simulink model "current_controller"  (R2015a)
settings: Solver=ode45  StartTime=0.0  StopTime=10.0  RelTol=1e-3
values from neighbouring files (symbols this model uses):
  Em = 115*sqrt(2)    [current_controller_param.m]
  Idref = 3    [current_controller_param.m]
  Iqref = 0    [current_controller_param.m]
  Kii = alphaI*R_hat    (= 628.318530718)    [VOC_param_paper.m]    (also in controller_parameters.m; current_controller_param.m = 1260)
  Kpi = alphaI*L_hat    (= 37.6991118431)    [VOC_param_paper.m]    (also in controller_parameters.m; current_controller_param.m = 62.8)
  L = 8e-3    (= 0.008)    [VOC_param.m]    (also in VOC_param_paper.m = 0.003; controller_parameters.m = 0.003; current_controller_param.m = 0.005; power_control_param.m)
  R = 0.1    [VOC_param.m]    (also in VOC_param_paper.m = 0.05; controller_parameters.m = 0.05; current_controller_param.m; power_control_param.m)
  w = 2*pi*f    (= 314.159265359)    [VOC_param.m]    (also in controller_parameters.m; current_controller_param.m; power_control_param.m)
libraries: powerlib_meascontrol x2, simulink x2
settings Model: Creator=rblan  LastModifiedBy=rblan

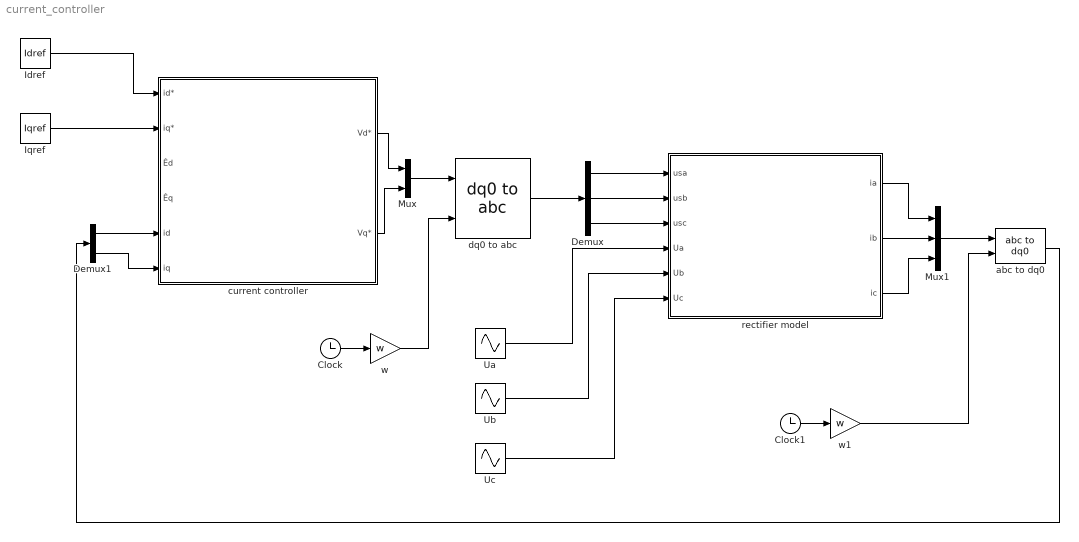
== system current_controller ==
  Clock : Clock
  Clock1 : Clock
  Demux : Demux  Outputs=3
  Demux1 : Demux  Outputs=2
  Idref : Constant  Value=Idref
  Iqref : Constant  Value=Iqref
  Mux : Mux  Inputs=2
  Mux1 : Mux  Inputs=3
  Ua : Sin  Amplitude=Em  Frequency=w  SampleTime=0
  Ub : Sin  Amplitude=Em  Frequency=w  Phase=-2*pi*3  SampleTime=0
  Uc : Sin  Amplitude=Em  Frequency=w  Phase=-4*pi/3  SampleTime=0
  abc to dq0 : powerlib_meascontrol/Transformations/abc to dq0  Alignment=90 degrees behind phase A axis
  "current controller " : Subsystem
  dq0 to abc : powerlib_meascontrol/Transformations/dq0 to abc  Alignment=90 degrees behind phase A axis
  rectifier model : Subsystem
  w : Gain  Gain=w
  w1 : Gain  Gain=w
  wires:
  "current controller "/1(Vd*) -> Mux/1
  "current controller "/2(Vq*) -> Mux/2
  Mux/1 -> dq0 to abc/1
  dq0 to abc/1 -> Demux/1
  Demux/1 -> rectifier model/1(usa)
  Demux/2 -> rectifier model/2(usb)
  Demux/3 -> rectifier model/3(usc)
  rectifier model/1(ia) -> Mux1/1
  rectifier model/2(ib) -> Mux1/2
  rectifier model/3(ic) -> Mux1/3
  Mux1/1 -> abc to dq0/1
  Demux1/2 -> "current controller "/6(iq)
  Demux1/1 -> "current controller "/5(id)
  abc to dq0/1 -> Demux1/1
  Ua/1 -> rectifier model/4(Ua)
  Ub/1 -> rectifier model/5(Ub)
  Uc/1 -> rectifier model/6(Uc)
  Idref/1 -> "current controller "/1(id*)
  Iqref/1 -> "current controller "/2(iq*)
  Clock/1 -> w/1
  w/1 -> dq0 to abc/2
  Clock1/1 -> w1/1
  w1/1 -> abc to dq0/2

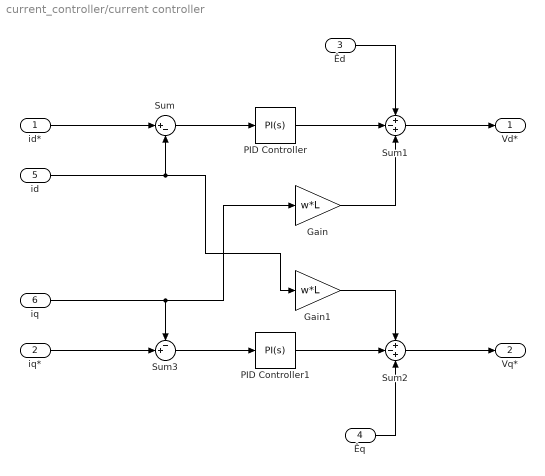
== system current_controller/current controller  ==
  id* : Inport
  iq* : Inport  Port=2
  Êd : Inport  Port=3
  Êq : Inport  Port=4
  id : Inport  Port=5
  iq : Inport  Port=6
  Gain : Gain  Gain=w*L
  Gain1 : Gain  Gain=w*L
  PID Controller : simulink/Continuous/PID Controller  Controller=PI  TimeDomain=Continuous-time  SampleTime=-1  IntegratorMethod=Forward Euler  FilterMethod=Forward Euler  Form=Parallel  UseFilter=on  ControllerParametersSource=internal  P=Kpi  I=Kii  D=0  N=100  InitialConditionSource=internal  InitialConditionForIntegrator=0  InitialConditionForFilter=0  ExternalReset=none  LimitOutput=off  UpperSaturationLimit=inf  LowerSaturationLimit=-inf  LinearizeAsGain=on  AntiWindupMode=none  Kb=1  TrackingMode=off  Kt=1  PParamMin=[]  PParamMax=[]  IParamMin=[]  IParamMax=[]  DParamMin=[]  DParamMax=[]  NParamMin=[]  NParamMax=[]  KbParamMin=[]  KbParamMax=[]  KtParamMin=[]  KtParamMax=[]  POutMin=[]  POutMax=[]  IOutMin=[]  IOutMax=[]  DOutMin=[]  DOutMax=[]  NOutMin=[]  NOutMax=[]  KbOutMin=[]  KbOutMax=[]  KtOutMin=[]  KtOutMax=[]  IntegratorOutMin=[]  IntegratorOutMax=[]  FilterOutMin=[]  FilterOutMax=[]  SumOutMin=[]  SumOutMax=[]  SumI1OutMin=[]  SumI1OutMax=[]  SumI2OutMin=[]  SumI2OutMax=[]  SumI3OutMin=[]  SumI3OutMax=[]  SumDOutMin=[]  SumDOutMax=[]  SaturationOutMin=[]  SaturationOutMax=[]  IntegratorContinuousStateAttributes=''  IntegratorStateMustResolveToSignalObject=off  IntegratorRTWStateStorageClass=Auto  FilterContinuousStateAttributes=''  FilterStateMustResolveToSignalObject=off  FilterRTWStateStorageClass=Auto  DifferentiatorICPrevScaledInput=0  DifferentiatorOutMin=[]  DifferentiatorOutMax=[]
  PID Controller1 : simulink/Continuous/PID Controller  Controller=PI  TimeDomain=Continuous-time  SampleTime=-1  IntegratorMethod=Forward Euler  FilterMethod=Forward Euler  Form=Parallel  UseFilter=on  ControllerParametersSource=internal  P=Kpi  I=Kii  D=0  N=100  InitialConditionSource=internal  InitialConditionForIntegrator=0  InitialConditionForFilter=0  ExternalReset=none  LimitOutput=off  UpperSaturationLimit=inf  LowerSaturationLimit=-inf  LinearizeAsGain=on  AntiWindupMode=none  Kb=1  TrackingMode=off  Kt=1  PParamMin=[]  PParamMax=[]  IParamMin=[]  IParamMax=[]  DParamMin=[]  DParamMax=[]  NParamMin=[]  NParamMax=[]  KbParamMin=[]  KbParamMax=[]  KtParamMin=[]  KtParamMax=[]  POutMin=[]  POutMax=[]  IOutMin=[]  IOutMax=[]  DOutMin=[]  DOutMax=[]  NOutMin=[]  NOutMax=[]  KbOutMin=[]  KbOutMax=[]  KtOutMin=[]  KtOutMax=[]  IntegratorOutMin=[]  IntegratorOutMax=[]  FilterOutMin=[]  FilterOutMax=[]  SumOutMin=[]  SumOutMax=[]  SumI1OutMin=[]  SumI1OutMax=[]  SumI2OutMin=[]  SumI2OutMax=[]  SumI3OutMin=[]  SumI3OutMax=[]  SumDOutMin=[]  SumDOutMax=[]  SaturationOutMin=[]  SaturationOutMax=[]  IntegratorContinuousStateAttributes=''  IntegratorStateMustResolveToSignalObject=off  IntegratorRTWStateStorageClass=Auto  FilterContinuousStateAttributes=''  FilterStateMustResolveToSignalObject=off  FilterRTWStateStorageClass=Auto  DifferentiatorICPrevScaledInput=0  DifferentiatorOutMin=[]  DifferentiatorOutMax=[]
  Sum : Sum  Inputs=|+-
  Sum1 : Sum  Inputs=+-+
  Sum2 : Sum  Inputs=+-+
  Sum3 : Sum  Inputs=-+|
  Vd* : Outport
  Vq* : Outport  Port=2
  wires:
  id*/1 -> Sum/1
  Sum/1 -> PID Controller/1
  PID Controller/1 -> Sum1/2
  Êd/1 -> Sum1/1
  Sum1/1 -> Vd*/1
  PID Controller1/1 -> Sum2/2
  Sum2/1 -> Vq*/1
  Êq/1 -> Sum2/3
  Sum3/1 -> PID Controller1/1
  iq*/1 -> Sum3/2
  id/1 -> Sum/2, Gain1/1
  iq/1 -> Gain/1, Sum3/1
  Gain/1 -> Sum1/3
  Gain1/1 -> Sum2/1

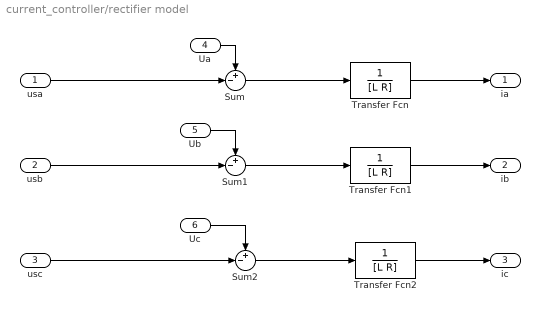
== system current_controller/rectifier model ==
  usa : Inport
  usb : Inport  Port=2
  usc : Inport  Port=3
  Ua : Inport  Port=4
  Ub : Inport  Port=5
  Uc : Inport  Port=6
  Sum : Sum  Inputs=+-|
  Sum1 : Sum  Inputs=+-|
  Sum2 : Sum  Inputs=+-|
  Transfer Fcn : TransferFcn  Denominator=[L R]
  Transfer Fcn1 : TransferFcn  Denominator=[L R]
  Transfer Fcn2 : TransferFcn  Denominator=[L R]
  ia : Outport
  ib : Outport  Port=2
  ic : Outport  Port=3
  wires:
  usa/1 -> Sum/2
  usc/1 -> Sum2/2
  Ua/1 -> Sum/1
  usb/1 -> Sum1/2
  Ub/1 -> Sum1/1
  Uc/1 -> Sum2/1
  Sum/1 -> Transfer Fcn/1
  Sum2/1 -> Transfer Fcn2/1
  Transfer Fcn/1 -> ia/1
  Transfer Fcn1/1 -> ib/1
  Sum1/1 -> Transfer Fcn1/1
  Transfer Fcn2/1 -> ic/1
